simulink model "mtpa_reference_test"  (R2015a)
settings: Solver=ode45  StartTime=0.0  StopTime=0.01  RelTol=1e-3
settings Model: Creator=user  LastModifiedBy=user

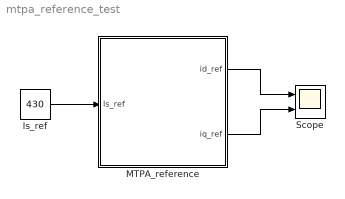
== system mtpa_reference_test ==
  Is_ref : Constant  Value=430
  MTPA_reference : MATLAB Function  TreatAsAtomicUnit=on
  Scope : Scope  NumInputPorts=2
      settings: YMin=-5~-5  YMax=5~5
  wires:
  Is_ref/1 -> MTPA_reference/1(Is_ref)
  MTPA_reference/1(id_ref) -> Scope/1
  MTPA_reference/2(iq_ref) -> Scope/2

== matlab function mtpa_reference_test/MTPA_reference ==
  data: Is_ref input; id_ref output; iq_ref output
function [id_ref, iq_ref] = MTPA_reference(Is_ref)

Ld = 0.090e-3;
Lq = 0.255e-3;
lambda_m = 0.0385;

DeltaL = Lq - Ld;

id_ref = (lambda_m - sqrt(lambda_m^2 + ...
          4*(DeltaL^2)*(Is_ref^2))) / (2*DeltaL);

iq_ref = sqrt(Is_ref^2 - id_ref^2);
